simulink model "DAB_IBDC_DPWM"  (R2019b)
settings: Solver=ode23t  StartTime=0.0  StopTime=0.1  RelTol=1e-3
libraries: powerlib x18, simulink x1
settings Model: Creator=khduh  LastModifiedBy=khduh

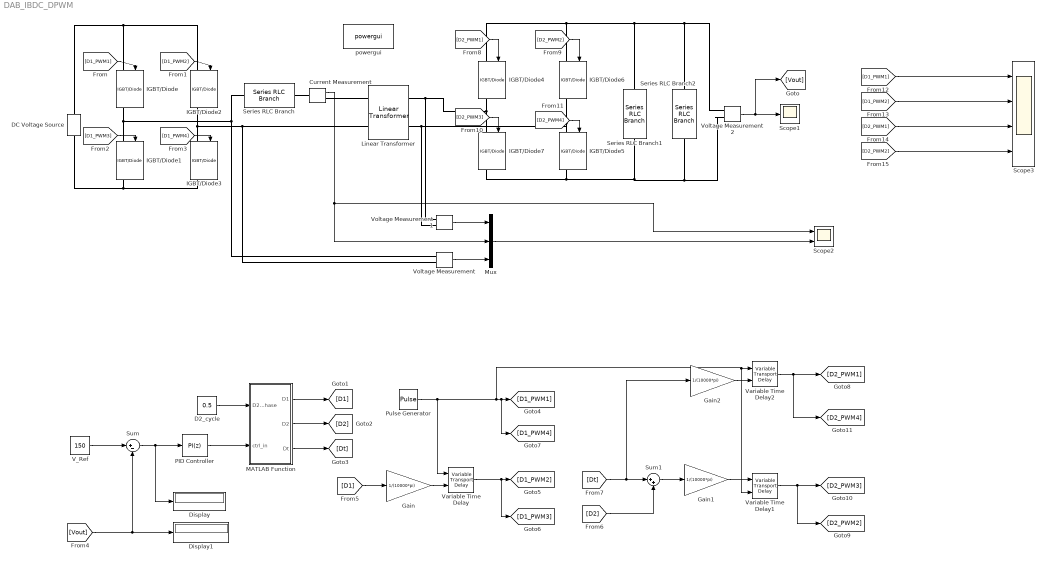
== system DAB_IBDC_DPWM ==
  Current Measurement : powerlib/Measurements/Current Measurement  PhasorSimulation=off  OutputType=Complex  PSBequivalent=0
      settings: SourceProductName=Simscape Electrical
  D2_cycle : Constant  Value=0.5
  DC Voltage Source : powerlib/Electrical Sources/DC Voltage Source  Amplitude=1000  Measurements=None
      settings: SourceProductName=Simscape Electrical
  Display : Display
  Display1 : Display
  Gain : Gain  Gain=1/(10000*pi)
  Gain1 : Gain  Gain=1/(10000*pi)
  Gain2 : Gain  Gain=1/(10000*pi)
  IGBT/Diode{,1..7} (8 alike) : powerlib/Power Electronics/IGBT//Diode  Ron=1e-3  Rs=1e5  Cs=inf  Measurements=on
      settings: SourceProductName=Simscape Electrical
  Linear Transformer : powerlib/Elements/Linear Transformer  UNITS=SI  NominalPower=[ 250e6 10000*pi ]  winding1=[500 0 0]  winding2=[250 0 0]  ThreeWindings=off  winding3=[3.15e+05 0.7938 0.084225]  RmLm=[1.0805e+06 2866]  Measurements=None  DataType=on
      settings: SourceProductName=Simscape Electrical
  MATLAB Function : MATLAB Function  TreatAsAtomicUnit=on
  Mux : Mux  Inputs=3
  PID Controller : simulink/Continuous/PID Controller  Controller=PI  Form=Parallel  TimeDomain=Discrete-time  SampleTime=-1  IntegratorMethod=Forward Euler  FilterMethod=Forward Euler  ControllerParametersSource=internal  P=.0000850  I=.25  D=0  UseFilter=on  N=100  TunerSelectOption=Transfer Function Based (PID Tuner App)  InitialConditionSource=internal  InitialConditionForIntegrator=0  InitialConditionForFilter=0  DifferentiatorICPrevScaledInput=0  ExternalReset=none  TrackingMode=off  Kt=1  LimitOutput=on  UpperSaturationLimit=.5  LowerSaturationLimit=-.5  LinearizeAsGain=on  AntiWindupMode=clamping  Kb=1  POutMin=[]  POutMax=[]  IOutMin=[]  IOutMax=[]  DOutMin=[]  DOutMax=[]  NOutMin=[]  NOutMax=[]  SumOutMin=[]  SumOutMax=[]  SaturationOutMin=[]  SaturationOutMax=[]  PParamMin=[]  PParamMax=[]  IParamMin=[]  IParamMax=[]  DParamMin=[]  DParamMax=[]  NParamMin=[]  NParamMax=[]  KbParamMin=[]  KbParamMax=[]  KtParamMin=[]  KtParamMax=[]  KbOutMin=[]  KbOutMax=[]  KtOutMin=[]  KtOutMax=[]  IntegratorOutMin=[]  IntegratorOutMax=[]  FilterOutMin=[]  FilterOutMax=[]  SumI1OutMin=[]  SumI1OutMax=[]  SumI2OutMin=[]  SumI2OutMax=[]  SumI3OutMin=[]  SumI3OutMax=[]  SumI4OutMin=[]  SumI4OutMax=[]  SumDOutMin=[]  SumDOutMax=[]  DifferentiatorOutMin=[]  DifferentiatorOutMax=[]  FilterDiffOutCoefMin=[]  FilterDiffOutCoefMax=[]  ReciprocalOutMin=[]  ReciprocalOutMax=[]  SumDenOutMin=[]  SumDenOutMax=[]  SumNumOutMin=[]  SumNumOutMax=[]  DivideOutMin=[]  DivideOutMax=[]  IntegratorContinuousStateAttributes=''  IntegratorStateMustResolveToSignalObject=off  IntegratorRTWStateStorageClass=Auto  FilterContinuousStateAttributes=''  FilterStateMustResolveToSignalObject=off  FilterRTWStateStorageClass=Auto  ParallelPVariant=InternalParameters  IdealPVariant=Disabled  IVariant=InternalParameters  DVariant=Disabled  IntegratorVariant=Discrete  SatVariant=Enabled  AWVariant=DiscClampingParallel  PCopyVariant=Disabled  TRVariant=Disabled  FdbkBlocksVariant=Forward  IdealPFdbkVariant=Disabled  SatFdbkVariant=Disabled  DerivativeFilterVariant=Disabled  NVariant=Disabled  NCopyVariant=Disabled_SignalSpec  FilterICVariant=Disabled  IntegratorICVariant=InternalICs  ExternalResetVariant=Disabled  TRSumVariant=Passthrough  SumFdbkVariant=Disabled  SumVariant=Sum_PI
  Pulse Generator : DiscretePulseGenerator  PulseType=Time based  Period=1/(10000*pi)  PulseWidth=50
  Scope1 : Scope
  Scope2 : Scope  NumInputPorts=2
  Scope3 : Scope  NumInputPorts=4
  Series RLC Branch : powerlib/Elements/Series RLC Branch  LConnTagsString=__new0  RConnTagsString=__new0  BranchType=L  Resistance=1  Inductance=.0102e-3  SetiL0=off  InitialCurrent=0  Capacitance=1e-6  Setx0=off  InitialVoltage=0  Measurements=None
      settings: SourceProductName=Simscape Electrical
  Series RLC Branch1 : powerlib/Elements/Series RLC Branch  LConnTagsString=__new0  RConnTagsString=__new0  BranchType=C  Resistance=1  Inductance=.0102e-3  SetiL0=off  InitialCurrent=0  Capacitance=660e-6  Setx0=off  InitialVoltage=0  Measurements=None
      settings: SourceProductName=Simscape Electrical
  Series RLC Branch2 : powerlib/Elements/Series RLC Branch  LConnTagsString=__new0  RConnTagsString=__new0  BranchType=R  Resistance=1  Inductance=.0102e-3  SetiL0=off  InitialCurrent=0  Capacitance=1e-6  Setx0=off  InitialVoltage=0  Measurements=None
      settings: SourceProductName=Simscape Electrical
  Sum : Sum  Inputs=|+-
  Sum1 : Sum  Inputs=|++
  V_Ref : Constant  Value=150
  Variable Time Delay : VariableTransportDelay  MaximumDelay=10
  Variable Time Delay1 : VariableTransportDelay  MaximumDelay=10
  Variable Time Delay2 : VariableTransportDelay  MaximumDelay=10
  Voltage Measurement : powerlib/Measurements/Voltage Measurement  PhasorSimulation=off  OutputType=Complex  PSBequivalent=0
      settings: SourceProductName=Simscape Electrical
  Voltage Measurement1 : powerlib/Measurements/Voltage Measurement  PhasorSimulation=off  OutputType=Complex  PSBequivalent=0
      settings: SourceProductName=Simscape Electrical
  Voltage Measurement2 : powerlib/Measurements/Voltage Measurement  PhasorSimulation=off  OutputType=Complex  PSBequivalent=0
      settings: SourceProductName=Simscape Electrical
  powergui : powerlib/powergui  Priority=1  SimulationMode=Discrete  SampleTime=1e-7  frequency=60  Iterations=50  frequencyindice=0  Pbase=100e6  ErrMax=1e-4  UnitsV=kV  UnitsW=MW  buscounter=0  FunctionMessages=off  echomessages=off  EnableUseOfTLC=off  CurrentSourceSwitches=off  DisableSnubberDevices=off  DisableRonSwitches=off  DisableVfSwitches=off  DisplayEquations=off  AutomaticDiscreteSolvers=off  SolverType=Tustin/Backward Euler (TBE)  Interpol=off  ExternalGateDelay=off  methode=off  Ts=100  x0status=blocks  SPID=on  SwTol=0  HookPort=off  NonlinearTolerance=1e-4  nMaxIteration=100  ContinueOnMaxIteration=off  RestoreLinks=warning  ResistiveCurrentMeasurement=off  Frange=[0:2:500]  Ylog=off  Xlog=on  ShowGrid=off  save=off  variable=ZData  structure=0  ZoomFFT=off  StartTime=0.0  cycles=1  DisplayStyle=1  fundamental=60  FreqAxis=off  MaxFrequency=1000  frequencyindicesteady=1  RmsSteady=1  display=off
      settings: SourceProductName=Simscape Electrical
  wires:
  Voltage Measurement/1 -> Mux/3
  Voltage Measurement1/1 -> Mux/1
  Voltage Measurement2/1 -> Scope1/1, [Vout]
  Current Measurement/1 -> Mux/2, Scope2/1
  [D1_PWM1] -> IGBT/Diode/1
  [D1_PWM2] -> IGBT/Diode2/1
  [D1_PWM3] -> IGBT/Diode1/1
  [D1_PWM4] -> IGBT/Diode3/1
  [Vout] -> Sum/2, Display1/1
  V_Ref/1 -> Sum/1
  MATLAB Function/1(D1) -> [D1]
  MATLAB Function/2(D2) -> [D2]
  MATLAB Function/3(Dt) -> [Dt]
  PID Controller/1 -> MATLAB Function/2(ctrl_in)
  Sum/1 -> PID Controller/1, Display/1
  D2_cycle/1 -> MATLAB Function/1(D2_phase)
  [D2_PWM3] -> IGBT/Diode7/1
  [D2_PWM1] -> IGBT/Diode4/1
  [D2_PWM2] -> IGBT/Diode6/1
  [D2_PWM4] -> IGBT/Diode5/1
  [D1] -> Gain/1
  Gain/1 -> Variable Time Delay/2
  Variable Time Delay/1 -> [D1_PWM3], [D1_PWM2]
  [Dt] -> Gain2/1, Sum1/1
  [D2] -> Sum1/2
  Sum1/1 -> Gain1/1
  Gain2/1 -> Variable Time Delay2/2
  Pulse Generator/1 -> Variable Time Delay/1, [D1_PWM4], [D1_PWM1], Variable Time Delay1/2, Variable Time Delay2/1
  Gain1/1 -> Variable Time Delay1/1
  Variable Time Delay2/1 -> [D2_PWM4], [D2_PWM1]
  Variable Time Delay1/1 -> [D2_PWM2], [D2_PWM3]
  Mux/1 -> Scope2/2
  [D1_PWM2] -> Scope3/2
  [D1_PWM1] -> Scope3/1
  [D2_PWM1] -> Scope3/3
  [D2_PWM2] -> Scope3/4
  connections:
  DC Voltage Source/LConn1 -- IGBT/Diode3/RConn1 -- IGBT/Diode1/RConn1
  IGBT/Diode1/LConn1 -- Series RLC Branch/LConn1 -- Voltage Measurement/LConn1 -- IGBT/Diode/RConn1
  IGBT/Diode2/RConn1 -- Voltage Measurement/LConn2 -- Linear Transformer/LConn2 -- IGBT/Diode3/LConn1
  DC Voltage Source/RConn1 -- IGBT/Diode/LConn1 -- IGBT/Diode2/LConn1
  Series RLC Branch/RConn1 -- Current Measurement/LConn1
  Current Measurement/RConn1 -- Linear Transformer/LConn1
  IGBT/Diode6/LConn1 -- Series RLC Branch1/RConn1 -- Series RLC Branch2/RConn1 -- Voltage Measurement2/LConn1 -- IGBT/Diode4/LConn1
  IGBT/Diode4/RConn1 -- Voltage Measurement1/LConn1 -- Linear Transformer/RConn1 -- IGBT/Diode7/LConn1
  IGBT/Diode5/LConn1 -- Voltage Measurement1/LConn2 -- Linear Transformer/RConn2 -- IGBT/Diode6/RConn1
  IGBT/Diode5/RConn1 -- Voltage Measurement2/LConn2 -- Series RLC Branch2/LConn1 -- Series RLC Branch1/LConn1 -- IGBT/Diode7/RConn1

== matlab function DAB_IBDC_DPWM/MATLAB Function ==
  data: D1 output; D2 output; Dt output; D2_phase input; ctrl_in input
function [D1,D2,Dt] = fcn(D2_phase,ctrl_in)
D2=D2_phase;
if 0<=D2_phase<=(ctrl_in+1/((ctrl_in^2)+ctrl_in+1))
    Dt=ctrl_in/(ctrl_in+1);
    D1=D2_phase*ctrl_in;
elseif (ctrl_in+1/((ctrl_in^2)+ctrl_in+1))<=D2_phase<=1
    Dt=ctrl_in/(ctrl_in+1);
    D1=1-(1/ctrl_in^2)+((1/ctrl_in^2)*D2_phase);
else
    D1=0;
    Dt=0;
    str="Error D2_phase is not between 0~1 "
    sprintf("%s",str)
end
